simulink model "12_1"  (R2018b)
settings: Solver=VariableStepAuto  StartTime=0  StopTime=10  MaxStep=0.001  RelTol=1e-3
InitFcn:
  | Bf = [2; 6];
  | a0 = -1;
  | a1 = 4;
  | b0 = -2;
  | b1 = 1;
  | w = 3^2;
  | w0 = 9.2/0.6;
  | Gamma = [0 1; -9 0];
  | 
  | syms k1 k2 k3 k4 k5;
  | eqn1 = k5 + a1 + k1*b1 == 5*w0;
  | eqn2 = w + a0 + k5*a1 + k1*b0 + k2*b1 == 10*w0^2;
  | eqn3 = k5*w + a1*w + k5*a0 + k2*b0 + k3*b1 == 10*w0^3;
  | eqn4 = a0*w + k3*b0 + k4*b1 + k5*a1*w == 5*w0^4;
  | eqn5 = k5*a0*w + k4*b0 == w0^5;
  | 
  | sol = solve([eqn1, eqn2, eqn3, eqn4, eqn5], [k1, k2, k3, k4, k5]);
  | K1 = double(sol.k1);
  | K2 = double(sol.k2);
  | K3 = double(sol.k3);
  | K4 = double(sol.k4);
  | K5 = double(sol.k5);
settings Model: Creator=kekos  LastModifiedBy=kekos

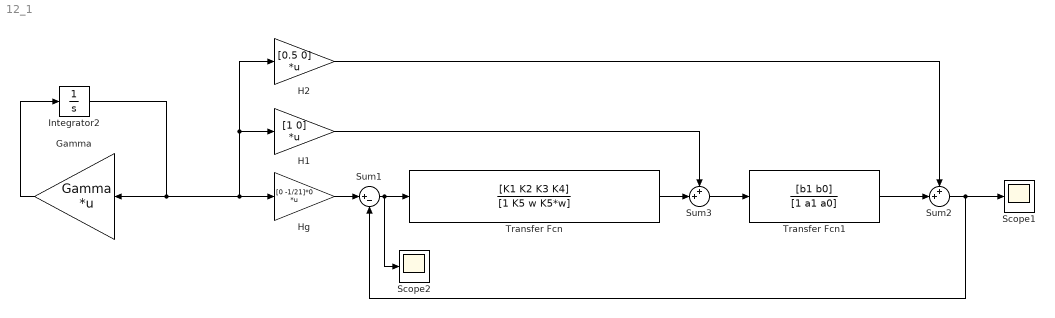
== system 12_1 ==
  Gamma : Gain  Gain=Gamma  Multiplication=Matrix(K*u)
  H1 : Gain  Gain=[1 0]  Multiplication=Matrix(K*u)
  H2 : Gain  Gain=[0.5 0]  Multiplication=Matrix(K*u)
  Hg : Gain  Gain=[0 -1/21]*0  Multiplication=Matrix(K*u)
  Integrator2 : Integrator  InitialCondition=[-2.91; -19.10]
  Scope1 : Scope
  Scope2 : Scope
  Sum1 : Sum  Inputs=|+-
  Sum2 : Sum  Inputs=++|
  Sum3 : Sum  Inputs=++|
  Transfer Fcn : TransferFcn  Numerator=[K1 K2 K3 K4]  Denominator=[1 K5 w K5*w]
  Transfer Fcn1 : TransferFcn  Numerator=[b1 b0]  Denominator=[1 a1 a0]
  wires:
  Gamma/1 -> Integrator2/1
  Hg/1 -> Sum1/1
  Sum1/1 -> Scope2/1, Transfer Fcn/1
  H2/1 -> Sum2/1
  Transfer Fcn/1 -> Sum3/2
  Sum3/1 -> Transfer Fcn1/1
  Transfer Fcn1/1 -> Sum2/2
  Sum2/1 -> Scope1/1, Sum1/2
  H1/1 -> Sum3/1
  Integrator2/1 -> H2/1, H1/1, Hg/1, Gamma/1
